simulink subsystem "guidance"  (R2024b)
settings: Solver=VariableStepAuto  StartTime=0.0  StopTime=10.0  RelTol=1e-3
settings Model: Creator=yagiz  LastModifiedBy=yagiz

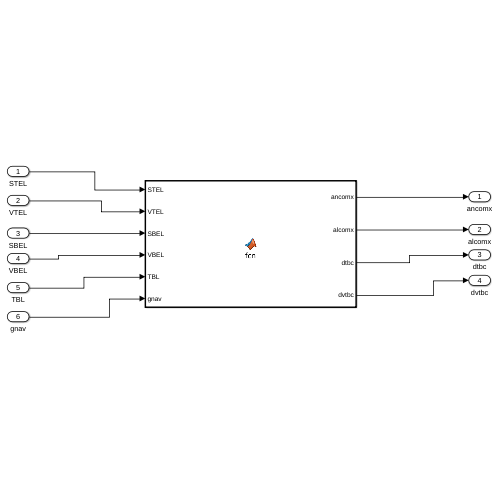
[thumbnail: Simulink's stored preview of the top-level diagram]
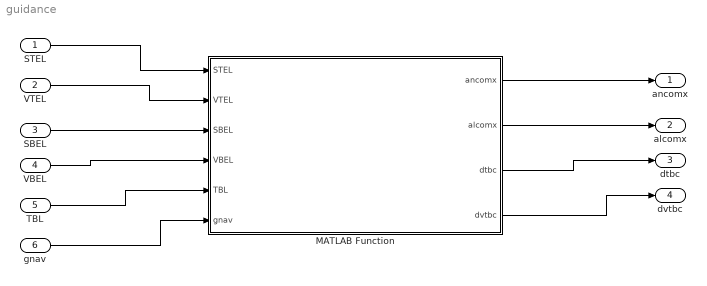
== system guidance ==
  STEL : Inport
  VTEL : Inport  Port=2
  SBEL : Inport  Port=3
  VBEL : Inport  Port=4
  TBL : Inport  Port=5
  gnav : Inport  Port=6
  MATLAB Function : MATLAB Function  TreatAsAtomicUnit=on
  ancomx : Outport
  alcomx : Outport  Port=2
  dtbc : Outport  Port=3
  dvtbc : Outport  Port=4
  wires:
  STEL/1 -> MATLAB Function/1(STEL)
  VTEL/1 -> MATLAB Function/2(VTEL)
  SBEL/1 -> MATLAB Function/3(SBEL)
  VBEL/1 -> MATLAB Function/4(VBEL)
  TBL/1 -> MATLAB Function/5(TBL)
  gnav/1 -> MATLAB Function/6(gnav)
  MATLAB Function/4(dvtbc) -> dvtbc/1
  MATLAB Function/3(dtbc) -> dtbc/1
  MATLAB Function/2(alcomx) -> alcomx/1
  MATLAB Function/1(ancomx) -> ancomx/1

== matlab function guidance/MATLAB Function ==
  data: STEL input; ancomx output; VTEL input; SBEL input; VBEL input; TBL input; gnav input; alcomx output; dtbc output; dvtbc output
function [ancomx, alcomx, dtbc, dvtbc] = fcn(STEL, VTEL, SBEL, VBEL, TBL, gnav)

AGRAV = 9.80665;
SMALL = 1e-7;

% LOS vector
STBLC = STEL - SBEL;
dtbc  = norm(STBLC);

if dtbc < SMALL
    ancomx = 0; alcomx = 0; dvtbc = 0;
    return;
end

UTBLC = STBLC / dtbc;

% Relative velocity
VTBLC = VTEL - VBEL;
dvtbc = abs(dot(UTBLC, VTBLC));

% LOS rate
WOELC = cross(UTBLC, VTBLC) / dtbc;

% Pro-Nav acceleration command (body axes, g's)
ACBX = TBL * cross(WOELC, UTBLC) * gnav * dvtbc / AGRAV;

% Limit
alimit = 50.0;
all_acc =  ACBX(2);
ann_acc = -ACBX(3);
aa = sqrt(all_acc^2 + ann_acc^2);
if aa > alimit
    phi    = atan2(ann_acc, all_acc);
    all_acc = alimit * cos(phi);
    ann_acc = alimit * sin(phi);
end

alcomx = all_acc;
ancomx = ann_acc;
